simulink model "QUESTION4_22"  (R2021a)
settings: Solver=VariableStepAuto  StartTime=0.0  StopTime=10.0  RelTol=1e-3
settings Model: Creator=user  LastModifiedBy=user

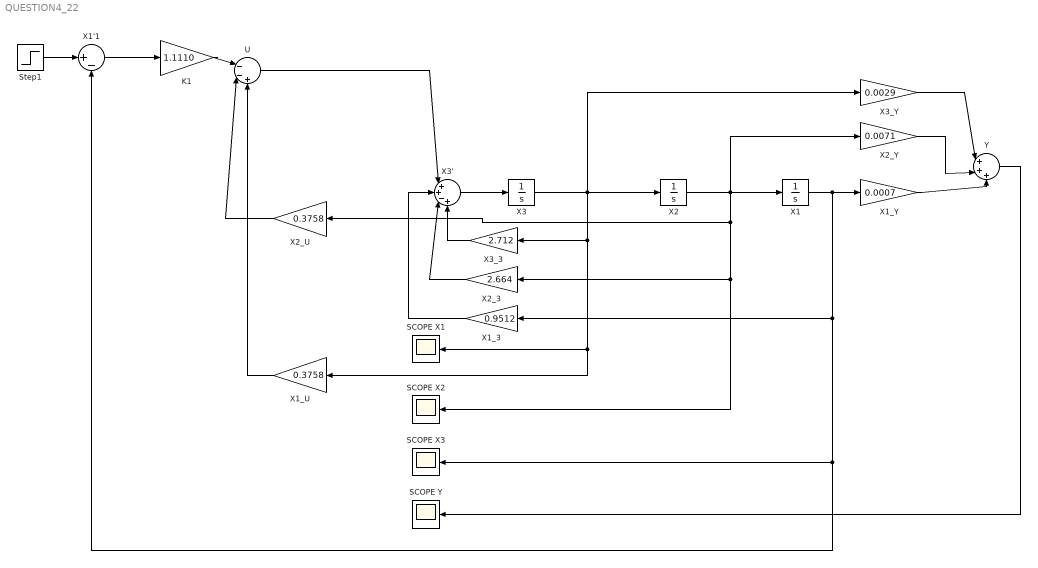
== system QUESTION4_22 ==
  K1 : Gain  Gain=1.1110
  SCOPE X1 : Scope
  SCOPE X2 : Scope
  SCOPE X3 : Scope
  SCOPE Y : Scope
  Step1 : Step  SampleTime=0
  U : Sum  Inputs=|--+
  X1 : Integrator
  X1'1 : Sum  Inputs=|+-
  X1_3 : Gain  Gain=0.9512
  X1_U : Gain  Gain=0.3758
  X1_Y : Gain  Gain=0.0007
  X2 : Integrator
  X2_3 : Gain  Gain=2.664
  X2_U : Gain  Gain=0.3758
  X2_Y : Gain  Gain=0.0071
  X3 : Integrator
  X3' : Sum  Inputs=|++-+
  X3_3 : Gain  Gain=2.712
  X3_Y : Gain  Gain=0.0029
  Y : Sum  Inputs=|+++
  wires:
  X1/1 -> X1_Y/1, X1_3/1, SCOPE X3/1, X1'1/2
  X3'/1 -> X3/1
  X1_Y/1 -> Y/3
  X2_Y/1 -> Y/2
  X3_Y/1 -> Y/1
  Y/1 -> SCOPE Y/1
  X1_3/1 -> X3'/2
  X2_3/1 -> X3'/3
  X3_3/1 -> X3'/4
  X2_U/1 -> U/2
  X1'1/1 -> K1/1
  K1/1 -> U/1
  X3/1 -> X3_3/1, SCOPE X1/1, X1_U/1, X3_Y/1, X2/1
  Step1/1 -> X1'1/1
  X2/1 -> X1/1, X2_Y/1, SCOPE X2/1, X2_3/1, X2_U/1
  X1_U/1 -> U/3
  U/1 -> X3'/1
